simulink model "SLAM_quad2"  (R2016a)
settings: Solver=FixedStepAuto  StartTime=0.0  StopTime=inf  FixedStep=0.01  RelTol=1e-3
model workspace (MAT data in the model file):
  SL_ROS_VariableLengthArrays_MaxSizes.CommonInfo.ArrayTruncateAction = 'EmitWarning'
  SL_ROS_VariableLengthArrays_MaxSizes.MsgTypeMap = containers.Map
  SL_ROS_VariableLengthArrays_MaxSizes.MsgTypeMap.serialization.keys = {'sensor_msgs/LaserScan'}
  SL_ROS_VariableLengthArrays_MaxSizes.MsgTypeMap.serialization.values{1}(1).PropertyName = 'Ranges'
  SL_ROS_VariableLengthArrays_MaxSizes.MsgTypeMap.serialization.values{1}(1).DataType = 'single'
  SL_ROS_VariableLengthArrays_MaxSizes.MsgTypeMap.serialization.values{1}(1).MaxLength = 180
  SL_ROS_VariableLengthArrays_MaxSizes.MsgTypeMap.serialization.values{1}(2).PropertyName = 'Intensities'
  SL_ROS_VariableLengthArrays_MaxSizes.MsgTypeMap.serialization.values{1}(2).DataType = 'single'
  SL_ROS_VariableLengthArrays_MaxSizes.MsgTypeMap.serialization.values{1}(2).MaxLength = 180
  SL_ROS_VariableLengthArrays_MaxSizes.MsgTypeMap.serialization.uniformity = 0
  SL_ROS_VariableLengthArrays_MaxSizes.MsgTypeMap.serialization.keyType = 'char'
  SL_ROS_VariableLengthArrays_MaxSizes.MsgTypeMap.serialization.valueType = 'any'
undefined symbols (not defined in the file): Header, Pose
libraries: robotlib x5, simulink x1
settings Model: Creator=UNIST  LastModifiedBy=UNIST
settings OptimizationCC: OptimizeModelRefInitCode=on  LifeSpan=Inf  MaxStackSize=64
settings HardwareCC: ProdBitPerPointer=32  ProdLargestAtomicFloat=None  ProdIntDivRoundTo=Undefined  ProdEndianess=Unspecified  ProdWordSize=32  ProdHWDeviceType=Generic->Unspecified (assume 32-bit Generic)
settings RTWCC: SystemTargetFile=ert.tlc  HardwareBoard=Robot Operating System (ROS)  TemplateMakefile=ert_default_tmf  GenerateReport=on  Toolchain=Catkin  IncludeHyperlinkInReport=on  LaunchReport=on  TargetLang=C++  GenerateTraceInfo=on  GenerateTraceReport=on  GenerateTraceReportSl=on  GenerateTraceReportSf=on  GenerateTraceReportEml=on
settings CodeAppCC: ForceParamTrailComments=on  IgnoreCustomStorageClasses=off  OperatorAnnotations=on  SimulinkDataObjDesc=on  SFDataObjDesc=on  MATLABFcnDesc=on  InsertBlockDesc=on  MATLABSourceComments=on
settings ERTTargetCC: SupportVariableSizeSignals=on

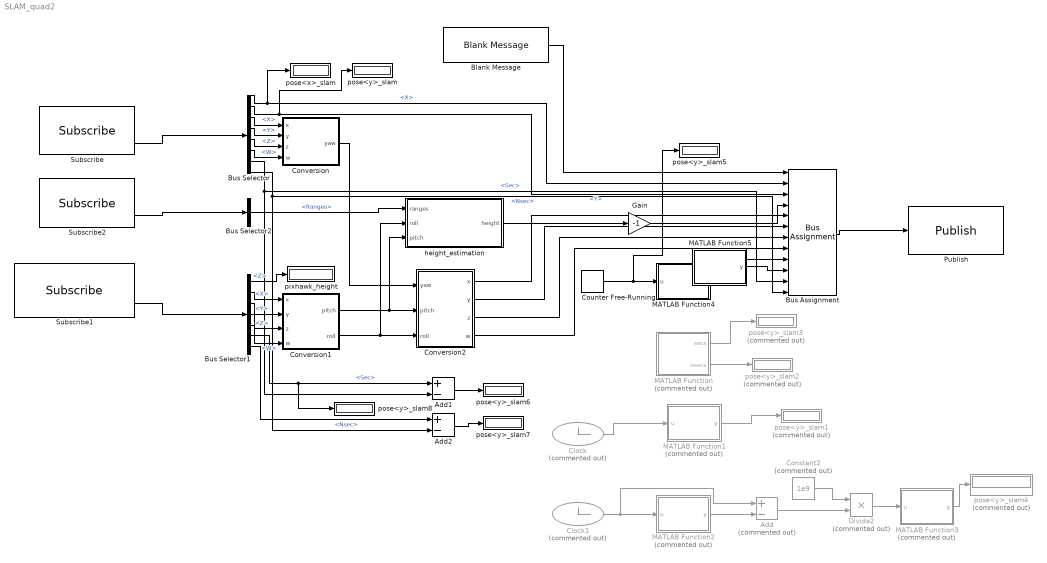
== system SLAM_quad2 ==
  Add : Sum  Commented=on  Inputs=+-
  Add1 : Sum  Inputs=+-
  Add2 : Sum  Inputs=+-
  Blank Message : robotlib/Blank Message  SourceLibraryInfo=This block requires Robotics System Toolbox  messageType=geometry_msgs/PoseStamped  SampleTime=-1
  Bus Assignment : BusAssignment  AssignedSignals=Pose.Position.X,Pose.Position.Y,Pose.Position.Z,Pose.Orientation.X,Pose.Orientation.Y,Pose.Orientation.Z,Pose.Orientation.W,Header.Seq,Header.FrameId,Header.Stamp.Sec,Header.Stamp.Nsec
  Bus Selector : BusSelector  OutputSignals=Pose.Pose.Position.X,Pose.Pose.Position.Y,Pose.Pose.Orientation.X,Pose.Pose.Orientation.Y,Pose.Pose.Orientation.Z,Pose.Pose.Orientation.W,Header.Stamp.Sec,Header.Stamp.Nsec
  Bus Selector1 : BusSelector  OutputSignals=Pose.Position.Z,Pose.Orientation.X,Pose.Orientation.Y,Pose.Orientation.Z,Pose.Orientation.W,Header.Stamp.Sec,Header.Stamp.Nsec
  Bus Selector2 : BusSelector  OutputSignals=Ranges
  Clock : Clock  Commented=on
  Clock1 : Clock  Commented=on
  Constant2 : Constant  Commented=on  Value=1e9
  Conversion : MATLAB Function  TreatAsAtomicUnit=on
  Conversion1 : MATLAB Function  TreatAsAtomicUnit=on
  Conversion2 : MATLAB Function  TreatAsAtomicUnit=on
  Counter Free-Running : simulink/Sources/Counter Free-Running  NumBits=16  tsamp=-1
  Divide2 : Product  Commented=on  Inputs=**
  Gain : Gain  Gain=-1
  MATLAB Function : MATLAB Function  Commented=on  TreatAsAtomicUnit=on
  MATLAB Function1 : MATLAB Function  Commented=on  TreatAsAtomicUnit=on
  MATLAB Function2 : MATLAB Function  Commented=on  TreatAsAtomicUnit=on
  MATLAB Function3 : MATLAB Function  Commented=on  TreatAsAtomicUnit=on
  MATLAB Function4 : MATLAB Function  TreatAsAtomicUnit=on
  MATLAB Function5 : MATLAB Function  TreatAsAtomicUnit=on
  Publish : robotlib/Publish  SourceLibraryInfo=This block requires Robotics System Toolbox  topicSource=Select from ROS network  topic=/mavros/vision_pose/pose  messageType=geometry_msgs/PoseStamped  messageQueueLength=1
  Subscribe : robotlib/Subscribe  SourceLibraryInfo=This block requires Robotics System Toolbox  topicSource=Select from ROS network  topic=/poseupdate  messageType=geometry_msgs/PoseWithCovarianceStamped  sampleTime=-1  messageQueueLength=1
  Subscribe1 : robotlib/Subscribe  SourceLibraryInfo=This block requires Robotics System Toolbox  topicSource=Select from ROS network  topic=/mavros/local_position/pose  messageType=geometry_msgs/PoseStamped  sampleTime=-1  messageQueueLength=1
  Subscribe2 : robotlib/Subscribe  SourceLibraryInfo=This block requires Robotics System Toolbox  topicSource=Select from ROS network  topic=/scan1  messageType=sensor_msgs/LaserScan  sampleTime=-1  messageQueueLength=1
  height_estimation : MATLAB Function  TreatAsAtomicUnit=on
  pixhawk_height : Display
  pose<x>_slam : Display
  pose<y>_slam{,5..8} (5 alike) : Display
  pose<y>_slam{1..4} (4 alike) : Display  Commented=on
  wires:
  Blank Message/1 -> Bus Assignment/1
  Bus Selector/1 -> Bus Assignment/2, pose<x>_slam/1  "<X>"
  Bus Selector/2 -> Bus Assignment/3, pose<y>_slam/1  "<Y>"
  Bus Selector1/1 -> pixhawk_height/1  "<Z>"
  Conversion/1(yaw) -> Conversion2/1(yaw)
  Conversion1/1(pitch) -> Conversion2/2(pitch), height_estimation/3(pitch)
  Conversion1/2(roll) -> Conversion2/3(roll), height_estimation/2(roll)
  Conversion2/1(x) -> Bus Assignment/5
  Conversion2/2(y) -> Bus Assignment/6
  Conversion2/3(z) -> Bus Assignment/7
  Conversion2/4(w) -> Bus Assignment/8
  Bus Selector/3 -> Conversion/1(x)  "<X>"
  Bus Selector/4 -> Conversion/2(y)  "<Y>"
  Bus Selector/5 -> Conversion/3(z)  "<Z>"
  Bus Selector/6 -> Conversion/4(w)  "<W>"
  Bus Selector1/2 -> Conversion1/1(x)  "<X>"
  Bus Selector1/3 -> Conversion1/2(y)  "<Y>"
  Bus Selector1/4 -> Conversion1/3(z)  "<Z>"
  Bus Selector1/5 -> Conversion1/4(w)  "<W>"
  Bus Selector2/1 -> height_estimation/1(ranges)  "<Ranges>"
  height_estimation/1(height) -> Gain/1
  Gain/1 -> Bus Assignment/4
  Subscribe1/2 -> Bus Selector1/1
  Subscribe2/2 -> Bus Selector2/1
  Subscribe/2 -> Bus Selector/1
  Bus Assignment/1 -> Publish/1
  Counter Free-Running/1 -> MATLAB Function4/1(u), pose<y>_slam5/1
  MATLAB Function4/1(y) -> Bus Assignment/9
  MATLAB Function1/1(y) -> pose<y>_slam1/1
  Clock1/1 -> MATLAB Function2/1(u), Add/1
  MATLAB Function2/1(y) -> Add/2
  Add/1 -> Divide2/2
  Constant2/1 -> Divide2/1
  Divide2/1 -> MATLAB Function3/1(u)
  MATLAB Function3/1(y) -> pose<y>_slam4/1
  Clock/1 -> MATLAB Function1/1(u)
  MATLAB Function/1(secs) -> pose<y>_slam3/1
  MATLAB Function/2(nsecs) -> pose<y>_slam2/1
  Bus Selector1/6 -> pose<y>_slam8/1, Add1/1  "<Sec>"
  Add1/1 -> pose<y>_slam6/1
  Bus Selector1/7 -> Add2/1  "<Nsec>"
  Add2/1 -> pose<y>_slam7/1
  Bus Selector/7 -> Bus Assignment/11, Add1/2  "<Sec>"
  Bus Selector/8 -> Bus Assignment/12, Add2/2  "<Nsec>"
  MATLAB Function5/1(y) -> Bus Assignment/10

== matlab function SLAM_quad2/Conversion1 ==
  data: pitch output; x input; y input; z input; w input; roll output
function [pitch,roll] = quat2eul(x,y,z,w)
%#codegen

% Convert the quaternion to a yaw angle (zyx euler angle)
eul = quat2eul([w,x,y,z]);
pitch = eul(2);
roll = eul(3);
end

== matlab function SLAM_quad2/Conversion ==
  data: yaw output; x input; y input; z input; w input
function yaw  = quat2eul(x,y,z,w)
%#codegen

% Convert the quaternion to a yaw angle (zyx euler angle)
eul = quat2eul([w,x,y,z]);
yaw = eul(1);

end

== matlab function SLAM_quad2/Conversion2 ==
  data: yaw input; pitch input; roll input; x output; y output; z output; w output
function [x,   y,   z,   w]   = eul2quat(yaw,pitch,roll)
%#codegen

% Convert the quaternion to a yaw angle (zyx euler angle)
q = eul2quat([yaw,pitch,roll]);
w=q(1);
x=q(2);
y=q(3);
z=q(4);
end

== matlab function SLAM_quad2/height_estimation ==
  data: ranges input; height output; roll input; pitch input
function height  = height_projection(ranges, roll, pitch)
    
    % get rid of errors from the mirror
    %mask = range < 0.12;
    %range(mask) = [];
%     if length(range)==0 return end
    % project the laser on the nomal vector of the floor
    ranges = double(ranges);
    height = mean(ranges) * cos(roll) * cos(pitch);
    height = height - 0.08;  % compansate the offset b/w mirror and laser

end

== matlab function SLAM_quad2/MATLAB Function ==
  data: secs output; nsecs output
function  [secs, nsecs] = fcn
%#codegen
secs = int32(0);
nsecs = int32(0);
coder.extrinsic('datetime', 'posixtime', 'now','datestr');
secs = int32(posixtime(datetime('now')));
nsecs = int32(str2double(datestr(now, 'FFF'))*1e6);

== matlab function SLAM_quad2/MATLAB Function1 ==
  data: u input; y output
function y = floor_1(u)
%#codegen

y = int32(floor(u));

== matlab function SLAM_quad2/MATLAB Function2 ==
  data: u input; y output
function y = floor_1(u)
%#codegen

y = floor(u);

== matlab function SLAM_quad2/MATLAB Function3 ==
  data: u input; y output
function y = floor_1(u)
%#codegen

y = int32(u);

== matlab function SLAM_quad2/MATLAB Function4 ==
  data: u input; y output
function y = double_1(u)
%#codegen

y = uint32(u);

== matlab function SLAM_quad2/MATLAB Function5 ==
  data: y output
function y = frame_id

y = uint8(1:128);
